simulink model "simplePI"  (R2018a)
settings: Solver=VariableStepAuto  StartTime=0.0  StopTime=10.0  RelTol=1e-3
undefined symbols (not defined in the file): ctl
settings Model: Creator=carca  LastModifiedBy=carca

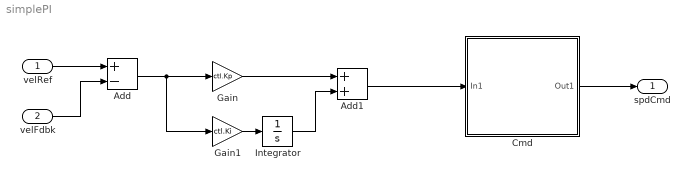
== system simplePI ==
  velRef : Inport
  velFdbk : Inport  Port=2
  Add : Sum  Inputs=+-
  Add1 : Sum
  Cmd : Subsystem
  Gain : Gain  Gain=ctl.Kp
  Gain1 : Gain  Gain=ctl.Ki
  Integrator : Integrator
  spdCmd : Outport
  wires:
  velRef/1 -> Add/1
  velFdbk/1 -> Add/2
  Add/1 -> Gain1/1, Gain/1
  Gain1/1 -> Integrator/1
  Gain/1 -> Add1/1
  Integrator/1 -> Add1/2
  Add1/1 -> Cmd/1(In1)
  Cmd/1(Out1) -> spdCmd/1

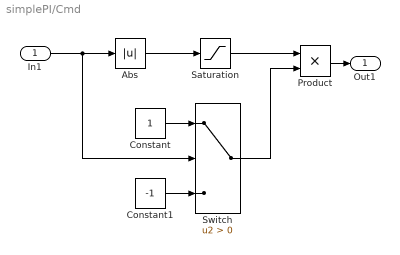
== system simplePI/Cmd ==
  In1 : Inport
  Abs : Abs
  Constant : Constant
  Constant1 : Constant  Value=-1
  Product : Product
  Saturation : Saturate  UpperLimit=1  LowerLimit=0
  Switch : Switch  Criteria=u2 > Threshold
  Out1 : Outport
  wires:
  Saturation/1 -> Product/1
  Abs/1 -> Saturation/1
  Switch/1 -> Product/2
  Constant1/1 -> Switch/3
  Product/1 -> Out1/1
  In1/1 -> Switch/2, Abs/1
  Constant/1 -> Switch/1
